simulink library "libControllers"  (R2015a)
settings: Solver=ode45  StartTime=0.0  StopTime=10.0  RelTol=1e-3
libraries: libControllers x1
settings Model: Creator=jcardena  LastModifiedBy=jcardena

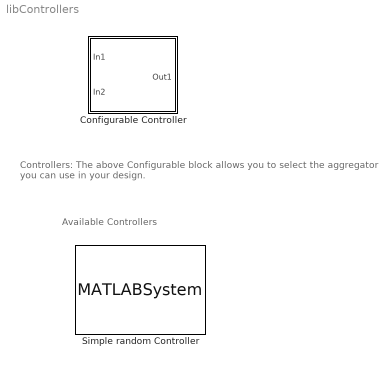
== system libControllers ==
  note: Available Controllers
  note: Controllers: The above Configurable block allows you to select the aggregator you can use in your design.
  Configurable Controller : Subsystem  BlockChoice=Simple random Controller
      settings: TemplateBlock=self  MemberBlocks=Simple random Controller
  Simple random Controller : MATLABSystem  System=db_Controller_mtlbSysBlock  db_name=HeatingUnits  db_username=sw_ETS  db_password=unb.sql.2015
      mask Type: db_Controller_mtlbSysBlock
      mask Display:
      | disp('Controller');
      | port_label('input',1,'aggIn');
      | port_label('input',2,'unitIDs');
      | port_label('output',1,'ctrlOut');

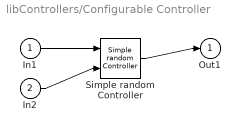
== system libControllers/Configurable Controller ==
  In1 : Inport
  In2 : Inport  Port=2
  Simple random Controller : libControllers/Simple random Controller  db_name=WaterHeaters  db_username=sw_waterheaters  db_password=unb.sql.2015
  Out1 : Outport
  wires:
  In1/1 -> Simple random Controller/1
  In2/1 -> Simple random Controller/2
  Simple random Controller/1 -> Out1/1
